simulink model "BPSK_demod"  (R2023b)
settings: Solver=ode45  StartTime=0.0  StopTime=20  MaxStep=0.01  MinStep=0.001  RelTol=1e-3  EnableMultiTasking=on
libraries: dspfdesign x3, simulink x1, simulink_extras x1
settings Model: Creator=SIMONA  LastModifiedBy=adiicmp_
settings SolverCC: AlgebraicLoopSolver=TrustRegion
settings DataIOCC: LimitDataPoints=on  SaveFormat=Array  ReturnWorkspaceOutputs=off
settings OptimizationCC: LifeSpan=inf
settings DebuggingCC: UnconnectedInputMsg=warning  UnconnectedOutputMsg=warning  UnconnectedLineMsg=warning  SFUnexpectedBacktrackingDiag=warning  SFNoUnconditionalDefaultTransitionDiag=warning  SFExecutionAtInitializationDiag=none  ArithmeticOperatorsInVariantConditions=warning
settings HardwareCC: ProdBitPerPointer=32  ProdBitPerSizeT=32  ProdBitPerPtrDiffT=32  ProdLargestAtomicFloat=None  ProdIntDivRoundTo=Undefined  ProdEndianess=Unspecified  ProdWordSize=32  ProdHWDeviceType=32-bit Generic
settings ModelReferenceCC: PropagateSignalLabelsOutOfModel=off
settings SFSimCC: SimUseLocalCustomCode=off  CustomCodeUndefinedFunction=UseInterfaceOnly
settings RTWCC: RTWUseLocalCustomCode=off
settings CodeAppCC: StateflowObjectComments=on
settings GRTTargetCC: TargetLangStandard=C89/C90 (ANSI)
settings ConfigComp: CovMetricSettings=dw  CovSaveCumulativeToWorkspaceVar=on  CovSaveSingleToWorkspaceVar=on  CovExternalEMLEnable=off

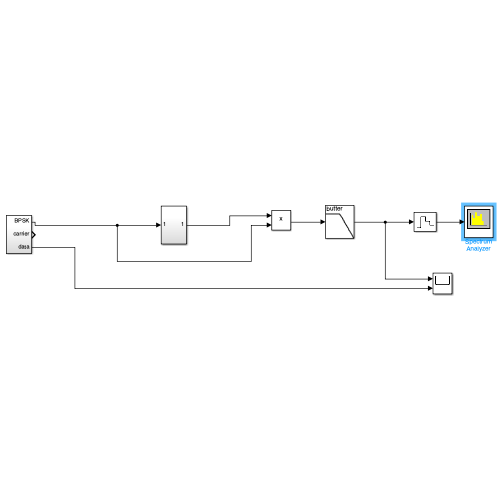
[thumbnail: Simulink's stored preview of the top-level diagram]
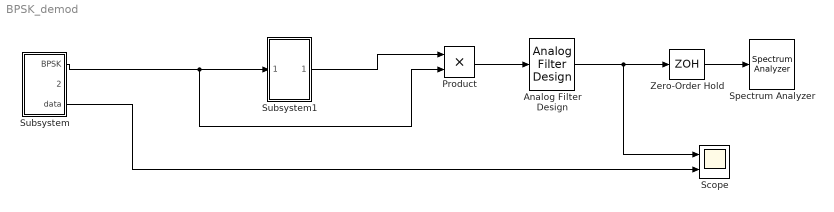
== system BPSK_demod ==
  Analog Filter Design : dspfdesign/Analog Filter Design  method=Butterworth  filttype=Lowpass  N=10  Wlo=pi*2*10  Whi=2*pi*2*10*(1+0.1)  Rp=2  Rs=40
  Product : Product
  Scope : Scope  NumInputPorts=2
  Spectrum Analyzer : SpectrumAnalyzer  WindowPosition=[320.000000,200.000000,800.000000,499.000000,]  ScopeFrameLocation=window  Span=100  StartFrequency=-50  StopFrequency=50  YLimits=[-3603.44492261,-2802.67938425]  SelectedToolstripTab=spectrumAnalyzerToolstrip.spectrumTab
  Subsystem : Subsystem
  Subsystem1 : Subsystem
  Zero-Order Hold : ZeroOrderHold  SampleTime=0.01
  wires:
  Subsystem/1(BPSK) -> Product/2, Subsystem1/1(In1)
  Subsystem1/1(Out2) -> Product/1
  Product/1 -> Analog Filter Design/1
  Analog Filter Design/1 -> Zero-Order Hold/1, Scope/1
  Subsystem/3(data) -> Scope/2
  Zero-Order Hold/1 -> Spectrum Analyzer/1

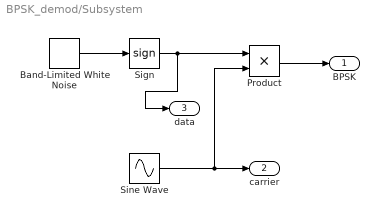
== system BPSK_demod/Subsystem ==
  Band-Limited White Noise : simulink/Sources/Band-Limited White Noise  Cov=[0.1]  Ts=1  seed=[23341]
  Product : Product
  Sign : Signum
  Sine Wave : Sin  Frequency=2*pi*10  SampleTime=0
  BPSK : Outport
  carrier : Outport  Port=2
  data : Outport  Port=3
  wires:
  Product/1 -> BPSK/1
  Sine Wave/1 -> Product/2, carrier/1
  Band-Limited White Noise/1 -> Sign/1
  Sign/1 -> data/1, Product/1

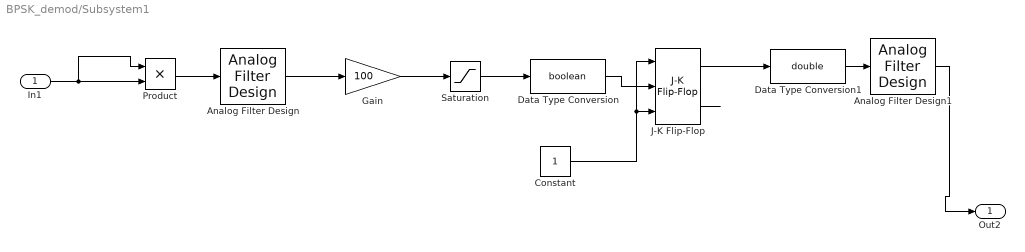
== system BPSK_demod/Subsystem1 ==
  In1 : Inport
  Analog Filter Design : dspfdesign/Analog Filter Design  method=Butterworth  filttype=Bandpass  N=10  Wlo=2*pi*2*10*(1-0.1)  Whi=2*pi*2*10*(1+0.1)  Rp=2  Rs=40
  Analog Filter Design1 : dspfdesign/Analog Filter Design  method=Butterworth  filttype=Bandpass  N=10  Wlo=pi*2*10*(1-0.1)  Whi=pi*2*10*(1+0.1)  Rp=2  Rs=40
  Constant : Constant  OutDataTypeStr=boolean
  Data Type Conversion : DataTypeConversion  OutDataTypeStr=boolean  SaturateOnIntegerOverflow=off  RndMeth=Floor
  Data Type Conversion1 : DataTypeConversion  OutDataTypeStr=double  SaturateOnIntegerOverflow=off  RndMeth=Floor
  Gain : Gain  Gain=100
  J-K Flip-Flop : simulink_extras/Flip Flops/J-K Flip-Flop  initial_condition=0
  Product : Product
  Saturation : Saturate  UpperLimit=1  LowerLimit=0
  Out2 : Outport
  wires:
  Gain/1 -> Saturation/1
  Analog Filter Design/1 -> Gain/1
  Saturation/1 -> Data Type Conversion/1
  In1/1 -> Product/1, Product/2
  Product/1 -> Analog Filter Design/1
  Data Type Conversion/1 -> J-K Flip-Flop/2
  Analog Filter Design1/1 -> Out2/1
  Data Type Conversion1/1 -> Analog Filter Design1/1
  Constant/1 -> J-K Flip-Flop/1, J-K Flip-Flop/3
  J-K Flip-Flop/1 -> Data Type Conversion1/1
  J-K Flip-Flop/2 -> ?
